simulink model "rths_tp9268dbfb_33ec_4127_aadf_5a8f8c5f2c47"  (R2025b)
settings: Solver=ode4  StartTime=0.0  StopTime=40  FixedStep=dt  RelTol=1e-3
model workspace (MAT data in the model file):
  A1 = [0 0 0 0 0 0 0 0 0 0 0 0 ... (900 elements, 30x30)]
  A2 = [0  0  0  0  0  0  1  0  0  0  0  0; 0  0  0  0  0  0  0  1  0  0  0  0; 0  0  0  0  0  0  0  0  1  0  0  0; 0  0  0  0  0  0  0  0  0  1  0  0; 0  0  0  0  0  0  0  0  0  0  1  0; 0  0  0  0  0  0  0  0  0  0  0  1; -10694.4349781  5856.94990807  -1040.71929003  11.5307208689  404.301043504  38.9379652927  -15.4601674269  7.74489325883  -1.37618725449  0.015247561227  0.534624416381  0.0514893228799; 5328.53946665  -7338.15654702  3271.075128  -395.655994048  -7.37150902836  305.73760326  7.04615372206  -11.0220181165  4.32548136925  -0.523192700845  -0.0097476590166  0.404289799235; -743.610380023  3117.65619945  -2550.3802986  -39.8797156523  -426.375336669  -346.26678026  -0.983307542293  4.12260901347  -4.69093853186  -0.0527346393203  -0.563814190411  -0.457883248839; 1198.47304489  -43070.3570903  -847.07354604  -47846.3421843  -10135.4030576  9.40762278729  1.58479173494  -56.9537598102  -1.12012127463  -64.5877099516  -13.4024733093  0.0124400985924; 40956.9002692  1865.86369803  -44643.302103  -10088.4890082  -47779.6872703  -10187.8449891  54.1590462232  2.46731069986  -59.0337317096  -13.340436872  -64.499569332  -13.4718194994; 4459.34545147  36448.3937635  -39559.0512001  -59.7609541575  -10144.1229091  -27367.227902  5.89678161296  48.1972568632  -52.3106111158  -0.0790244441664  -13.4140039387  -37.5073086094]
  A3 = [0 0 0 0 0 0 0 0 0 -11216.7436102 6120.49164694 -1250.45258802 ... (324 elements, 18x18)]
  B1 = [0  0  0  0  0  0  0  0  0  0  0  0  0  0  0; 0  0  0  0  0  0  0  0  0  0  0  0  0  0  0; 0  0  0  0  0  0  0  0  0  0  0  0  0  0  0; 0  0  0  0  0  0  0  0  0  0  0  0  0  0  0; 0  0  0  0  0  0  0  0  0  0  0  0  0  0  0; 0  0  0  0  0  0  0  0  0  0  0  0  0  0  0; 0  0  0  0  0  0  0  0  0  0  0  0  0  0  0; 0  0  0  0  0  0  0  0  0  0  0  0  0  0  0; 0  0  0  0  0  0  0  0  0  0  0  0  0  0  0; 0  0  0  0  0  0  0  0  0  0  0  0  0  0  0; 0  0  0  0  0  0  0  0  0  0  0  0  0  0  0; 0  0  0  0  0  0  0  0  0  0  0  0  0  0  0; 0  0  0  0  0  0  0  0  0  0  0  0  0  0  0; 0  0  0  0  0  0  0  0  0  0  0  0  0  0  0; 0  0  0  0  0  0  0  0  0  0  0  0  0  0  0; 0.000162210458758  0  0  0  0  0  0  0  0  0  0  0  0  0  0; 0  0.0195741403137  0  0  0  0  0  0  0  0  0  0  0  0  0; 0  0  0.0147303099554  0  0  0  0  0  0  0  0  0  0  0  0; 0  0  0  0.0147303099554  0  0  0  0  0  0  0  0  0  0  0; 0  0  0  0  0.0195741403137  0  0  0  0  0  0  0  0  0  0; 0  0  0  0  0  0.000162210458758  0  0  0  0  0  0  0  0  0; 0  0  0  0  0  0  0.0195741403137  0  0  0  0  0  0  0  0; 0  0  0  0  0  0  0  0.0147303099554  0  0  0  0  0  0  0; 0  0  0  0  0  0  0  0  0.0147303099554  0  0  0  0  0  0; 0  0  0  0  0  0  0  0  0  0.0195741403137  0  0  0  0  0; 0  0  0  0  0  0  0  0  0  0  0.000162210458758  0  0  0  0; 0  0  0  0  0  0  0  0  0  0  0  0.0195741403137  0  0  0; 0  0  0  0  0  0  0  0  0  0  0  0  0.0147303099554  0  0; 0  0  0  0  0  0  0  0  0  0  0  0  0  0.0147303099554  0; 0  0  0  0  0  0  0  0  0  0  0  0  0  0  0.0195741403137]
  B2 = [0  0  0  0  0  0; 0  0  0  0  0  0; 0  0  0  0  0  0; 0  0  0  0  0  0; 0  0  0  0  0  0; 0  0  0  0  0  0; 0.000155509146218  3.03510417428e-06  1.08758134818e-06  -6.78354563204e-06  1.77315145951e-05  -1.45419663101e-05; 3.03510417428e-06  0.000145654356285  1.02904123458e-05  -8.79437622207e-06  -7.79542878529e-06  3.49356219206e-05; 1.08758134818e-06  1.02904123458e-05  0.000151423071674  1.63543431294e-06  -3.16589562281e-06  -2.55082053341e-05; -6.78354563204e-06  -8.79437622207e-06  1.63543431294e-06  0.0146724361839  2.91102137942e-05  -2.16951142623e-05; 1.77315145951e-05  -7.79542878529e-06  -3.16589562281e-06  2.91102137942e-05  0.0146543064443  6.59348973663e-05; -1.45419663101e-05  3.49356219206e-05  -2.55082053341e-05  -2.16951142623e-05  6.59348973663e-05  0.0145485119653]
  B3 = [0  0  0  0  0  0  0  0  0; 0  0  0  0  0  0  0  0  0; 0  0  0  0  0  0  0  0  0; 0  0  0  0  0  0  0  0  0; 0  0  0  0  0  0  0  0  0; 0  0  0  0  0  0  0  0  0; 0  0  0  0  0  0  0  0  0; 0  0  0  0  0  0  0  0  0; 0  0  0  0  0  0  0  0  0; 0.000159186201117  -2.54024240345e-06  4.65575255871e-06  -2.40646746724e-06  8.1196183977e-06  4.37381616231e-06  0.000302935336269  0.00126264599362  0.00156203975266; -2.54024240345e-06  0.000154107993859  4.88016101925e-06  -1.54311353769e-05  6.77864041829e-06  6.25450457057e-06  -0.000459326699367  -0.00191449113814  -0.0023684479094; 4.65575255871e-06  4.88016101925e-06  0.000154885583422  5.88289993993e-06  -1.24931676457e-05  -7.15255052644e-06  0.000293964918962  0.00122525695339  0.0015157851671; -2.40646746724e-06  -1.54311353769e-05  5.88289993993e-06  0.014680380812  1.08842148256e-05  1.49205088267e-05  0.001698259817  0.00213312637172  0.0011075391107; 8.1196183977e-06  6.77864041829e-06  -1.24931676457e-05  1.08842148256e-05  0.0146962651234  -1.84930265115e-05  -0.00411085573378  -0.00486398973958  -0.00221765410407; 4.37381616231e-06  6.25450457057e-06  -7.15255052644e-06  1.49205088267e-05  -1.84930265115e-05  0.0147185175842  0.00845575577146  0.00974441342285  0.0041586471669; 0.000302935336269  -0.000459326699367  0.000293964918962  0.001698259817  -0.00411085573378  0.00845575577146  1.00869498175  0.0176088889684  0.016014507749; 0.00126264599362  -0.00191449113814  0.00122525695339  0.00213312637172  -0.00486398973958  0.00974441342285  0.0176088889684  1.05175826224  0.057330972257; 0.00156203975266  -0.0023684479094  0.0015157851671  0.0011075391107  -0.00221765410407  0.0041586471669  0.016014507749  0.057330972257  1.06800860627]
  C1 = [1  0  0  0  0  0  0  0  0  0  0  0  0  0  0  0  0  0  0  0  0  0  0  0  0  0  0  0  0  0; 0  0  0  0  0  1  0  0  0  0  0  0  0  0  0  0  0  0  0  0  0  0  0  0  0  0  0  0  0  0; 0  0  0  0  0  0  0  0  0  0  1  0  0  0  0  0  0  0  0  0  0  0  0  0  0  0  0  0  0  0]
  C2 = [1  0  0  0  0  0  0  0  0  0  0  0; 0  1  0  0  0  0  0  0  0  0  0  0; 0  0  1  0  0  0  0  0  0  0  0  0]
  C3 = [1  0  0  0  0  0  0  0  0  0  0  0  0  0  0  0  0  0; 0  1  0  0  0  0  0  0  0  0  0  0  0  0  0  0  0  0; 0  0  1  0  0  0  0  0  0  0  0  0  0  0  0  0  0  0]
  D1 = [0  0  0  0  0  0  0  0  0  0  0  0  0  0  0; 0  0  0  0  0  0  0  0  0  0  0  0  0  0  0; 0  0  0  0  0  0  0  0  0  0  0  0  0  0  0]
  D2 = [0  0  0  0  0  0; 0  0  0  0  0  0; 0  0  0  0  0  0]
  D3 = [0  0  0  0  0  0  0  0  0; 0  0  0  0  0  0  0  0  0; 0  0  0  0  0  0  0  0  0]
  cb_force = [6164.83060128; 6164.83060128; 6164.83060128; 0; 0; 0; 0; 0; 0]
  dt = 0.0009765625
  excitation_input = [0 0.0009765625 0.001953125 0.0029296875 0.00390625 0.0048828125 0.005859375 0.0068359375 0.0078125 0.0087890625 0.009765625 0.0107421875 ... (81922 elements, 40961x2)]
  full_force = [6164.83060128; 0; 0; 0; 0; 6164.83060128; 0; 0; 0; 0; 6164.83060128; 0; 0; 0; 0]
  guyan_force = [6164.83060128; 6164.83060128; 6164.83060128; 0; 0; 0]
settings Model: Creator=lenovo  LastModifiedBy=lenovo
settings DataIOCC: SaveOutput=off  SignalLogging=off  SaveTime=off

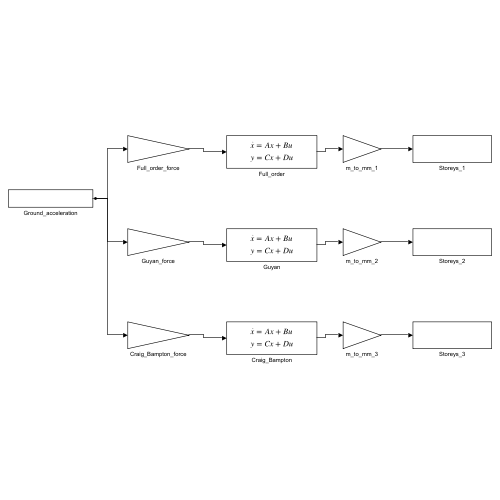
[thumbnail: Simulink's stored preview of the top-level diagram]
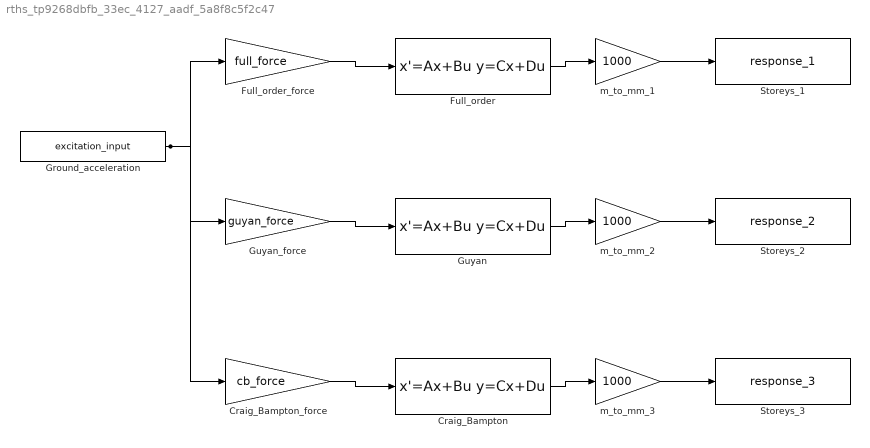
== system rths_tp9268dbfb_33ec_4127_aadf_5a8f8c5f2c47 ==
  Craig_Bampton : StateSpace  A=A3  B=B3  C=C3  D=D3  InitialCondition=0
  Craig_Bampton_force : Gain  Gain=cb_force
  Full_order : StateSpace  A=A1  B=B1  C=C1  D=D1  InitialCondition=0
  Full_order_force : Gain  Gain=full_force
  Ground_acceleration : FromWorkspace  VariableName=excitation_input  OutputAfterFinalValue=Holding final value
  Guyan : StateSpace  A=A2  B=B2  C=C2  D=D2  InitialCondition=0
  Guyan_force : Gain  Gain=guyan_force
  Storeys_1 : ToWorkspace  VariableName=response_1  SaveFormat=Timeseries  SampleTime=-1
  Storeys_2 : ToWorkspace  VariableName=response_2  SaveFormat=Timeseries  SampleTime=-1
  Storeys_3 : ToWorkspace  VariableName=response_3  SaveFormat=Timeseries  SampleTime=-1
  m_to_mm_1 : Gain  Gain=1000
  m_to_mm_2 : Gain  Gain=1000
  m_to_mm_3 : Gain  Gain=1000
  wires:
  Ground_acceleration/1 -> Full_order_force/1, Guyan_force/1, Craig_Bampton_force/1
  Full_order_force/1 -> Full_order/1
  Full_order/1 -> m_to_mm_1/1
  m_to_mm_1/1 -> Storeys_1/1
  Guyan_force/1 -> Guyan/1
  Guyan/1 -> m_to_mm_2/1
  m_to_mm_2/1 -> Storeys_2/1
  Craig_Bampton_force/1 -> Craig_Bampton/1
  Craig_Bampton/1 -> m_to_mm_3/1
  m_to_mm_3/1 -> Storeys_3/1
